simulink model "TestSP"  (Simulink 8.5)
settings: Solver=ode45  StartTime=0.0  StopTime=10.0  RelTol=1e-3
settings Model: Creator=Dr.Ranjith  LastModifiedBy=admin  CovSFcnEnable=off
settings DataIOCC: SignalLoggingSaveFormat=Dataset
settings OptimizationCC: ExpressionDepthLimit=128
settings DebuggingCC: UnderspecifiedInitializationDetection=Simplified  MergeDetectMultiDrivingBlocksExec=error  SolverPrmCheckMsg=warning  FcnCallInpInsideContextMsg=EnableAllAsError  StateNameClashWarn=none
settings GRTTargetCC: CombineOutputUpdateFcns=on  GRTInterface=off

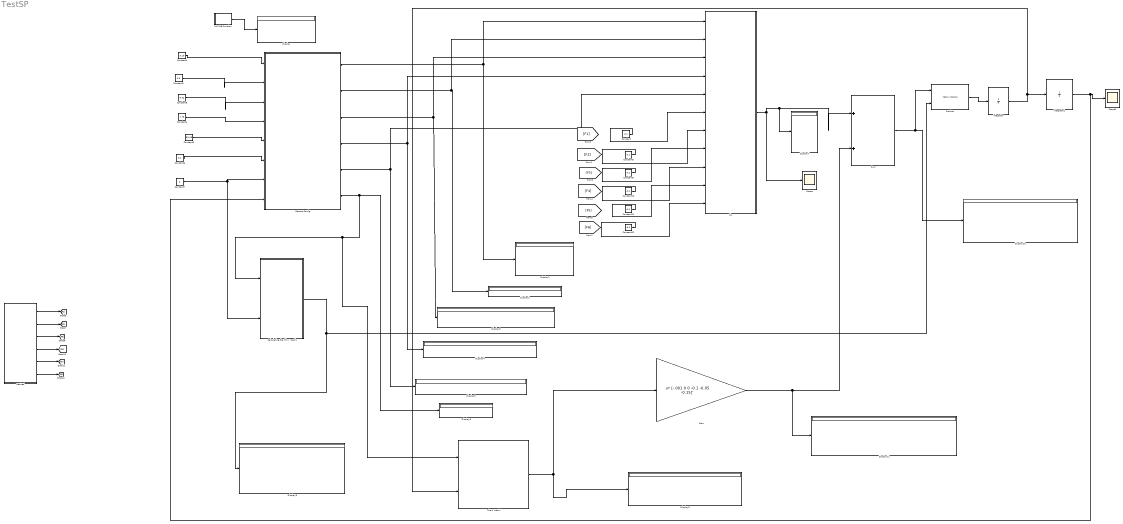
== system TestSP ==
  Calculating the Minv  matrix : MATLAB Function  TreatAsAtomicUnit=on
  Constant : Constant  Value=0.1
  Constant1 : Constant  Value=0.10
  Constant10 : Constant  Value=-0.1
  Constant11 : Constant  Value=-0.1
  Constant12 : Constant  Value=-0.1
  Constant2 : Constant  Value=0.3
  Constant3 : Constant  Value=0.02
  Constant4 : Constant  Value=7.75
  Constant5 : Constant  Value=53.45
  Constant6 : Constant  Value=0.2
  Constant7 : Constant  Value=2
  Constant8 : Constant  Value=0.1
  Constant9 : Constant  Value=0.1
  Desired : Subsystem
  Display{,1..11} (12 alike) : Display
  Gain : Gain  Gain=[-.001 0 0 -0.1 -0.05 -0.15]'  Multiplication=Matrix(u*K)
  Integrator : Integrator
  Integrator1 : Integrator
  MATLAB Function : MATLAB Function  TreatAsAtomicUnit=on
  Product : Product  Multiplication=Matrix(*)
  Scope : Scope
  Scope1 : Scope
  Stewart Config : MATLAB Function  TreatAsAtomicUnit=on
  Sum : Sum  Inputs=|++
  The H matrix : MATLAB Function  TreatAsAtomicUnit=on
  Uin : MATLAB Function  TreatAsAtomicUnit=on
  wires:
  ? -> MATLAB Function/1(a)
  MATLAB Function/1(b) -> Display/1
  Constant1/1 -> Stewart Config/1(rp)
  Constant2/1 -> Stewart Config/2(rb)
  Constant3/1 -> Stewart Config/3(hp)
  Constant4/1 -> Stewart Config/4(gammap1)
  Constant5/1 -> Stewart Config/5(gammab1)
  Constant6/1 -> Stewart Config/6(vert)
  Constant7/1 -> Calculating the Minv  matrix/2(mplatform), Stewart Config/7(mplatform)
  Stewart Config/6(bIp) -> The H matrix/1(bIp), Calculating the Minv  matrix/1(bIp), Display6/1
  Stewart Config/3(bb) -> Uin/3(bb), Display3/1
  Stewart Config/2(bdp) -> Uin/2(bdp), Display2/1
  Constant/1 -> Uin/6(F1)
  Constant8/1 -> Uin/7(F2)
  Constant9/1 -> Uin/8(F3)
  Constant10/1 -> Uin/9(F4)
  Stewart Config/5(bA) -> Uin/5(bA), Display5/1
  Stewart Config/4(pp) -> Display4/1, Uin/4(pp)
  Constant11/1 -> Uin/10(F5)
  Constant12/1 -> Uin/11(F6)
  Stewart Config/1(bRp) -> Display1/1, Uin/1(bRp)
  Calculating the Minv  matrix/1(Minv) -> Product/2, Display8/1
  Desired/1(F1) -> [F1]
  Desired/5(F5) -> [F5]
  Desired/4(F4) -> [F4]
  Desired/6(F6) -> [F6]
  Desired/2(F2) -> [F2]
  Desired/3(F3) -> [F3]
  The H matrix/1(H) -> Display9/1, Gain/1
  Gain/1 -> Display11/1, Sum/2
  Integrator1/1 -> Stewart Config/8(X), Scope1/1
  Sum/1 -> Product/1, Display10/1
  Uin/1(Uin) -> Scope/1, Display7/1, Sum/1
  Product/1 -> Integrator/1
  Integrator/1 -> The H matrix/2(Xdot), Integrator1/1

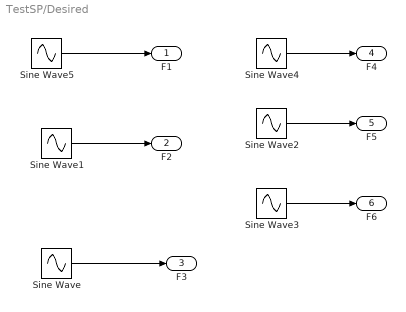
== system TestSP/Desired ==
  Sine Wave : Sin  Amplitude=0.29  Frequency=0.6283  SampleTime=0
  Sine Wave1 : Sin  Amplitude=0.3  Frequency=0.628  Phase=1.57  SampleTime=0
  Sine Wave2 : Sin  Amplitude=0.305  Frequency=0.6283  SampleTime=0
  Sine Wave3 : Sin  Amplitude=0.28  Frequency=0.6283  Phase=1.57  SampleTime=0
  Sine Wave4 : Sin  Amplitude=0.31  Frequency=0.6283  Phase=1.57  SampleTime=0
  Sine Wave5 : Sin  Amplitude=0.3  Frequency=0.628  SampleTime=0
  F1 : Outport
  F2 : Outport  Port=2
  F3 : Outport  Port=3
  F4 : Outport  Port=4
  F5 : Outport  Port=5
  F6 : Outport  Port=6
  wires:
  Sine Wave/1 -> F3/1
  Sine Wave1/1 -> F2/1
  Sine Wave5/1 -> F1/1
  Sine Wave2/1 -> F5/1
  Sine Wave3/1 -> F6/1
  Sine Wave4/1 -> F4/1

== matlab function Stewart Config ==
  data: rp input double; bRp output double; rb input double; hp input double; gammap1 input double; gammab1 input double; vert input double; mplatform input double; bdp output double; bb output double; pp output double; bA output double; bIp output double; X input double
function [bRp,bdp,bb,pp,bA,bIp] = fcn(rp,rb,hp,gammap1,gammab1,vert,mplatform,X)
%#codegen
%The states that were chosen were X=[x,y,z,phi,theta,psi] and
%X2=[xdot,ydot,zdot,p,q,r ]
%Due to this a  trnasformation matrix must be added to transform the body
%rates to Euler rates.
gammap = [gammap1,120-gammap1, 120+gammap1, -120-gammap1,-120+gammap1,-gammap1];
gammab = [gammab1,120-gammab1, 120+gammab1, -120-gammab1,-120+gammab1,-gammab1];

 %alphap = [0 , 120, 120, -120 , -120 , 0] ;  
 %betab = [60,60,180,180,-60,-60];
 

 % pIp = mplatform *[((rp^2)/4) , 0, 0; 0, ((rp*2)/4), 0; 0, 0, (rp^2)/2] ;
    pp=zeros(3,6);
    pp(1,: ) = rp*cos(gammap*pi/180);
    pp(2,: ) = rp*sin(gammap*pi/180) ;
    pp(3,: ) = [hp/2,hp/2,hp/2,hp/2,hp/2,hp/2 ] ;        %hp is the thickness of the platform
    bb=zeros(3,6);
    bb(1,: ) = rb*cos(gammab*pi/180);
    bb(2,: ) = rb*sin(gammab*pi/180);
    bb(3,: ) = [0 , 0, 0, 0 , 0, 0] ;
    
     bdp = [X(1,a),X(2,a),X(3,a)+vert]' ;                       %Position of platform frame wrt base
     %bdp=[0.01,0.02,0.03+vert]';
    bDp = [bdp,bdp,bdp,bdp,bdp,bdp] ;                           %This is same for all 6 actuators
   
      psi=X(4,a);
      the=X(5,a);
      phi=X(6,a);
    %psi=0.0872;
    %the=0;
    %phi=0;
    
   
    spsi = sin(psi);
    cpsi = cos(psi);
    sthe = sin(the);
    cthe = cos(the);
    sphi = sin(phi);
    cphi = cos(phi);
    

    
    pIp = mplatform *[((0.15^2)/4) , 0, 0; 0, ((0.15*2)/4), 0; 0, 0, (0.15^2)/2] ;
    bRp=zeros(3,3);
    bRp(1,1 ) = cphi * cthe ;
    bRp(1,2 ) = -sphi*cpsi + cphi * sthe * spsi ;
    bRp(1,3 ) = sphi * spsi + cphi * sthe * cpsi ;
    bRp(2,1 ) = sphi * cthe ;
    bRp(2,2 ) = cphi * cpsi + sphi * sthe * spsi ;
    bRp(2,3 ) = -cphi * spsi + sphi * sthe * cpsi ;
    bRp(3,1 ) = -sthe ;
    bRp(3,2 ) = cthe * spsi ;
    bRp(3,3 ) = cthe * cpsi ;
    
     bA = bRp*pp + bDp - bb ;                                    %Actuator vector
    
     bIp=bRp*pIp*bRp';                                           %Inertia tensor varying due to orientation of platform wrt base
end

== matlab function MATLAB Function ==
  data: a input double; b output double
function b = fcn(a)
%#codegen
b=zeros(3,3);
for i=1:3
for j=1:3
    b(i,j)=a+i+j;
end
end

end

== matlab function Uin ==
  data: bRp input double; bdp input double; bb input double; Uin output double; pp input double; bA input double; F1 input double; F2 input double; F3 input double; F4 input double; F5 input double; F6 input double
function Uin = fcn(bRp,bdp,bb,pp,bA,F1,F2,F3,F4,F5,F6)
%#codegen
    g=9.81;
    G=[0,0,-g]';
    Fvec=zeros(3,6);
    %We are going to add g in vector form to the input force
   %Uin=zeros(6,1);
    %for j=1:6
     %  Fvec(:,j)=F(j,a)*bA(:,j);
    %end
    Fvec(:,1)=F1*bA(:,1);
    Fvec(:,2)=F2*bA(:,2);
    Fvec(:,3)=F3*bA(:,3);
    Fvec(:,4)=F4*bA(:,4);
    Fvec(:,5)=F5*bA(:,5);
    Fvec(:,6)=F6*bA(:,6);
      
    
   U=zeros(6,1);                                              %Combined effect of gravity and force on actuators
     %for j=1:6
      % U(j,1)= F(j,a)+dot(Fvec(:,j),G);
     %end
     
     
     U(1,1)=F1+dot(Fvec(:,1),G);
     U(2,1)=F2+dot(Fvec(:,2),G);
     U(3,1)=F3+dot(Fvec(:,3),G);
     U(4,1)=F4+dot(Fvec(:,4),G);
     U(5,1)=F5+dot(Fvec(:,5),G);
     U(6,1)=F6+dot(Fvec(:,6),G);
    
     Jt=zeros(6,6);
   
      for i=1:6
      Jt(:,i ) = [ ( bRp*pp(:,i) + bdp - bb(:,i) ); cross( bRp*pp(:,i),bdp-bb(:,i) ) ] / norm(bA(:,i)) ;
  
      end
    
     Uin=Jt*U;                                                %Input u in state space form
end

== matlab function Calculating the Minv  matrix ==
  data: bIp input double; mplatform input double; Minv output double
function Minv = fcn(bIp,mplatform)
%#codegen
%Minv=zeros(6,6);
m=mplatform*(eye(3));

z=zeros(3,3);
M=zeros(6,6);
Minv=zeros(6,6);
M=[m,z;z,bIp];
Minv=inv(M);
end

== matlab function The H matrix ==
  data: bIp input double; H output double; Xdot input double
function H = fcn(bIp,Xdot)
%#codegen
%H=zeros(6,6);
bWp = [Xdot(4,1) ; Xdot(5,1) ; Xdot(6,1)] ;
%bWp=[0.1;0.05;0.15];
bWpskew=zeros(3,3);
bWpskew=[ 0 , -1*bWp(3,1) , bWp(2,1) ; 
         bWp(3,1) , 0 , -1*bWp(1,1)  ;
         -1*bWp(2,1), bWp(1,1), 0 ];
     z=zeros(3,3);
     h=zeros(3,3);
     h= bWpskew*bIp;                             %WxI 
    H=[z,z;z,h];
